simulink library "dlbsBlockSpecifyDimensions"  (R2025b)
settings: Solver=VariableStepAuto  StartTime=0.0  StopTime=10.0  RelTol=1e-3
libraries: dlbsBlockExtractGradientGF x1, dlbsBlockInsertGradientGF x1
settings Model: Creator=lt6037  LastModifiedBy=lt6037

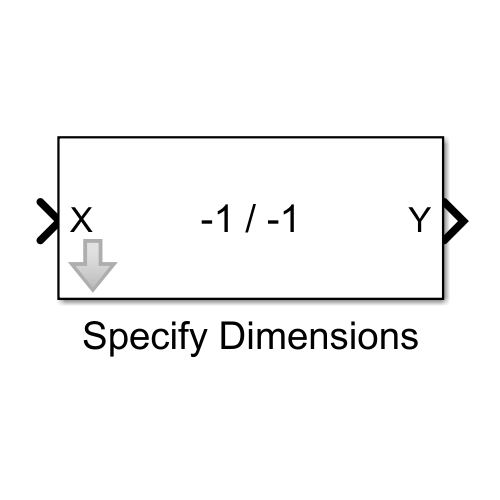
[thumbnail: Simulink's stored preview of the top-level diagram]
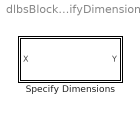
== system dlbsBlockSpecifyDimensions ==
  Specify Dimensions : Subsystem  mask{value_size=-1, grad_size=-1}
      mask prompts: value_size "Value size"; grad_size "Gradient size"
      mask help:
      | Passes the input value through while explicitly constraining value and gradient signal dimensions.
      | This block is useful for debugging and for stabilizing signal width propagation in Simulink models.
      mask Help: web("dlbsHelpBlockSpecifyDimensions.html")
      mask Display:
      | s = [...
      |     "Spec Dims",...
      |     sprintf("Value: %s",get_param(gcb,"value_size")),...
      |     sprintf("Grad: %s",get_param(gcb,"grad_size")),...
      |     ];
      | 
      | % fprintf(join(s,"\n"))
      | 
      | 
      | fprintf("%s / %s",get_param(gcb,"value_size"),get_param(gcb,"grad_size"))

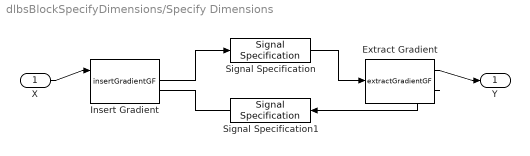
== system dlbsBlockSpecifyDimensions/Specify Dimensions ==
  X : Inport
  Extract Gradient : dlbsBlockExtractGradientGF/extractGradientGF
  Insert Gradient : dlbsBlockInsertGradientGF/insertGradientGF
  Signal Specification : SignalSpecification  Dimensions=value_size
  Signal Specification1 : SignalSpecification  Dimensions=grad_size
  Y : Outport
  wires:
  Extract Gradient/2 -> Signal Specification1/1
  Insert Gradient/1 -> Signal Specification/1
  Signal Specification/1 -> Extract Gradient/1
  Signal Specification1/1 -> Insert Gradient/2
  X/1 -> Insert Gradient/1
  Extract Gradient/1 -> Y/1
